simulink model "Lazoabierto_urinario22"  (R2023a)
settings: Solver=ode15s  StartTime=0.0  StopTime=10.0  MaxStep=1e-3  RelTol=1e-3
settings Model: Creator=najap  LastModifiedBy=DELL
settings DataIOCC: ReturnWorkspaceOutputs=off  TimeSaveName=t
settings DebuggingCC: AlgebraicLoopMsg=none  ArtificialAlgebraicLoopMsg=none  MaxConsecutiveZCsMsg=none  ModelReferenceExtraNoncontSigs=none  OperatingPointInterfaceChecksumMismatchMsg=none

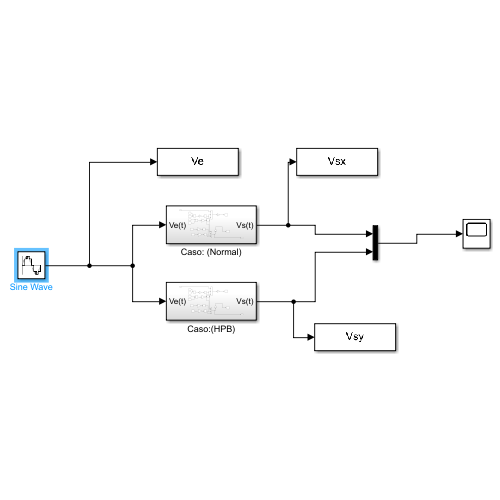
[thumbnail: Simulink's stored preview of the top-level diagram]
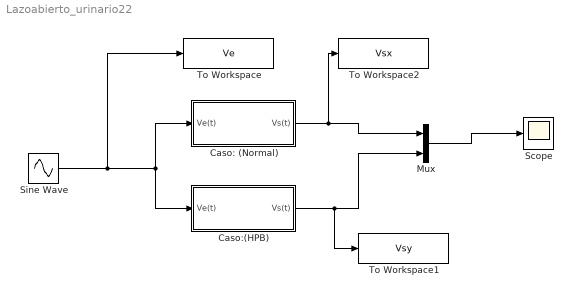
== system Lazoabierto_urinario22 ==
  Caso: (Normal) : Subsystem
  Caso:(HPB) : Subsystem
  Mux : Mux  Inputs=2
  Scope : Scope
  Sine Wave : Sin  Amplitude=8  Frequency=1.5708  SampleTime=0.001
  To Workspace : ToWorkspace  VariableName=Ve  SaveFormat=Timeseries  SampleTime=-1
  To Workspace1 : ToWorkspace  VariableName=Vsy  SaveFormat=Timeseries  SampleTime=-1
  To Workspace2 : ToWorkspace  VariableName=Vsx  SaveFormat=Timeseries  SampleTime=-1
  wires:
  Sine Wave/1 -> To Workspace/1, Caso: (Normal)/1(Ve(t)), Caso:(HPB)/1(Ve(t))
  Mux/1 -> Scope/1
  Caso:(HPB)/1(Vs(t)) -> To Workspace1/1, Mux/2
  Caso: (Normal)/1(Vs(t)) -> To Workspace2/1, Mux/1

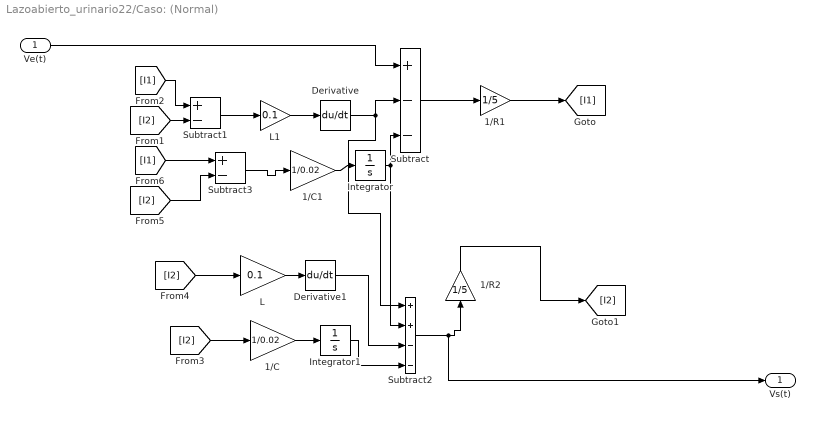
== system Lazoabierto_urinario22/Caso: (Normal) ==
  Ve(t) : Inport
  1/C : Gain  Gain=1/0.02
  1/C1 : Gain  Gain=1/0.02
  1/R1 : Gain  Gain=1/5
  1/R2 : Gain  Gain=1/5
  Derivative : Derivative
  Derivative1 : Derivative
  Integrator : Integrator
  Integrator1 : Integrator
  L : Gain  Gain=0.1
  L1 : Gain  Gain=0.1
  Subtract : Sum  Inputs=+--
  Subtract1 : Sum  Inputs=+-
  Subtract2 : Sum  Inputs=++--
  Subtract3 : Sum  Inputs=+-
  Vs(t) : Outport
  wires:
  [I2] -> L/1
  Ve(t)/1 -> Subtract/1
  Subtract3/1 -> 1/C1/1
  Subtract2/1 -> Vs(t)/1, 1/R2/1
  Subtract1/1 -> L1/1
  [I1] -> Subtract1/1
  [I2] -> Subtract1/2
  [I2] -> Subtract3/2
  [I1] -> Subtract3/1
  1/R2/1 -> [I2]
  Derivative/1 -> Subtract/2, Subtract2/1
  L1/1 -> Derivative/1
  1/C1/1 -> Integrator/1
  Integrator/1 -> Subtract/3, Subtract2/2
  Subtract/1 -> 1/R1/1
  1/R1/1 -> [I1]
  L/1 -> Derivative1/1
  Derivative1/1 -> Subtract2/3
  [I2] -> 1/C/1
  Integrator1/1 -> Subtract2/4
  1/C/1 -> Integrator1/1

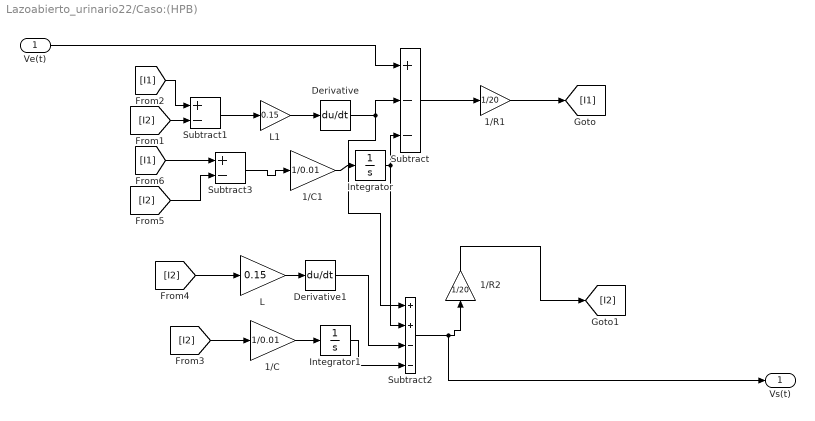
== system Lazoabierto_urinario22/Caso:(HPB) ==
  Ve(t) : Inport
  1/C : Gain  Gain=1/0.01
  1/C1 : Gain  Gain=1/0.01
  1/R1 : Gain  Gain=1/20
  1/R2 : Gain  Gain=1/20
  Derivative : Derivative
  Derivative1 : Derivative
  Integrator : Integrator
  Integrator1 : Integrator
  L : Gain  Gain=0.15
  L1 : Gain  Gain=0.15
  Subtract : Sum  Inputs=+--
  Subtract1 : Sum  Inputs=+-
  Subtract2 : Sum  Inputs=++--
  Subtract3 : Sum  Inputs=+-
  Vs(t) : Outport
  wires:
  L/1 -> Derivative1/1
  Derivative1/1 -> Subtract2/3
  1/C/1 -> Integrator1/1
  Integrator1/1 -> Subtract2/4
  Subtract/1 -> 1/R1/1
  1/R2/1 -> [I2]
  Derivative/1 -> Subtract/2, Subtract2/1
  [I2] -> 1/C/1
  1/C1/1 -> Integrator/1
  1/R1/1 -> [I1]
  L1/1 -> Derivative/1
  [I2] -> L/1
  Integrator/1 -> Subtract/3, Subtract2/2
  Subtract1/1 -> L1/1
  Ve(t)/1 -> Subtract/1
  [I2] -> Subtract1/2
  Subtract3/1 -> 1/C1/1
  Subtract2/1 -> Vs(t)/1, 1/R2/1
  [I1] -> Subtract1/1
  [I2] -> Subtract3/2
  [I1] -> Subtract3/1
